simulink model "PSK"  (R2016a)
settings: Solver=FixedStepDiscrete  StartTime=0.0  StopTime=0.05  FixedStep=1/2000000  RelTol=1e-3
libraries: dspsigops x2, dsparch4 x2
settings Model: Creator=camj3302  LastModifiedBy=camj3302

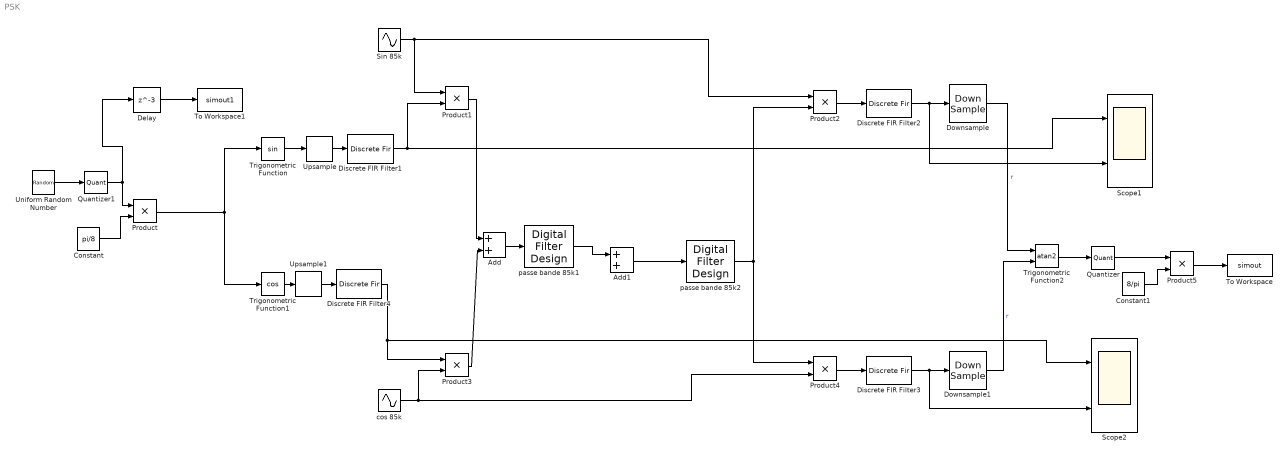
== system PSK ==
  Add : Sum
  Add1 : Sum
  Constant : Constant  Value=pi/8  SampleTime=1/1000
  Constant1 : Constant  Value=8/pi  SampleTime=1/1000
  Delay : Delay  DelayLength=3  InitialCondition=0
  Discrete FIR Filter{1..4} (4 alike) : DiscreteFir  Coefficients=sin([0:1999]/1999*pi)
  Downsample : DownSample  N=2000  RateOptions=Allow multirate processing
  Downsample1 : DownSample  N=2000  RateOptions=Allow multirate processing
  Product{,1..5} (6 alike) : Product
  Quantizer : Quantizer  QuantizationInterval=pi/8
  Quantizer1 : Quantizer  QuantizationInterval=1
  Scope1 : Scope  NumInputPorts=2
  Scope2 : Scope  NumInputPorts=2
  Sin 85k : Sin  Frequency=85000*2*pi  SampleTime=1/2000000
  To Workspace : ToWorkspace  VariableName=simout  SampleTime=-1
      settings: Save2DSignal=2-D array (concatenate along first dimension)
  To Workspace1 : ToWorkspace  VariableName=simout1  SampleTime=-1
      settings: Save2DSignal=2-D array (concatenate along first dimension)
  Trigonometric Function : Trigonometry
  Trigonometric Function1 : Trigonometry  Operator=cos
  Trigonometric Function2 : Trigonometry  Operator=atan2  ApproximationMethod=CORDIC
  Uniform Random Number : UniformRandomNumber  Minimum=0  Maximum=15  SampleTime=1/1000
  Upsample : dspsigops/Upsample  N=2000  phase=0  RateOptions=Allow multirate processing  ic=0  mode=Unused parameter value
  Upsample1 : dspsigops/Upsample  N=2000  phase=0  RateOptions=Allow multirate processing  ic=0  mode=Unused parameter value
  cos 85k : Sin  Frequency=85000*2*pi  Phase=pi/2  SampleTime=1/2000000
  passe bande 85k1 : dsparch4/Digital Filter Design  mwdsp_browser_bugfix_var=off
  passe bande 85k2 : dsparch4/Digital Filter Design  mwdsp_browser_bugfix_var=off
  wires:
  Product2/1 -> Discrete FIR Filter2/1
  Sin 85k/1 -> Product1/1, Product2/1
  Product1/1 -> Add/1
  Add/1 -> passe bande 85k1/1
  Discrete FIR Filter2/1 -> Downsample/1, Scope1/2
  Product4/1 -> Discrete FIR Filter3/1
  cos 85k/1 -> Product3/2, Product4/2
  passe bande 85k2/1 -> Product4/1, Product2/2
  Product3/1 -> Add/2
  Discrete FIR Filter3/1 -> Downsample1/1, Scope2/2
  Downsample1/1 -> Trigonometric Function2/2  "r"
  Downsample/1 -> Trigonometric Function2/1  "r"
  Trigonometric Function2/1 -> Quantizer/1
  Uniform Random Number/1 -> Quantizer1/1
  Constant/1 -> Product/2
  Add1/1 -> passe bande 85k2/1
  passe bande 85k1/1 -> Add1/1
  Trigonometric Function/1 -> Upsample/1
  Trigonometric Function1/1 -> Upsample1/1
  Product/1 -> Trigonometric Function1/1, Trigonometric Function/1
  Constant1/1 -> Product5/2
  Quantizer1/1 -> Delay/1, Product/1
  Quantizer/1 -> Product5/1
  Product5/1 -> To Workspace/1
  Delay/1 -> To Workspace1/1
  Upsample/1 -> Discrete FIR Filter1/1
  Discrete FIR Filter1/1 -> Product1/2, Scope1/1
  Discrete FIR Filter4/1 -> Scope2/1, Product3/1
  Upsample1/1 -> Discrete FIR Filter4/1
